simulink model "Lab1"  (R2016a)
settings: Solver=VariableStepAuto  StartTime=0.0  StopTime=10.0  RelTol=1e-3
settings Model: Creator=KamalEldeen  LastModifiedBy=KamalEldeen

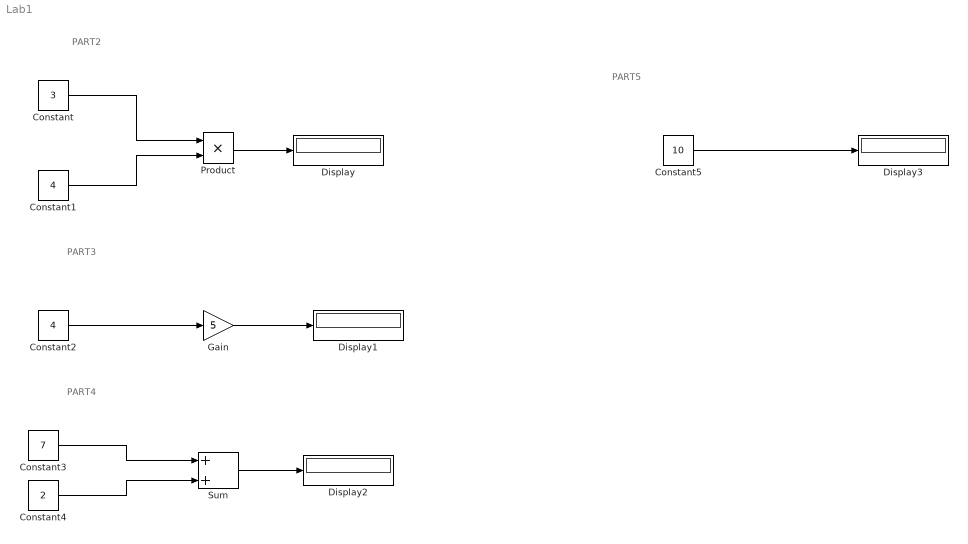
== system Lab1 ==
  note: PART2
  note: PART3
  note: PART4
  note: PART5
  Constant : Constant  Value=3
  Constant1 : Constant  Value=4
  Constant2 : Constant  Value=4
  Constant3 : Constant  Value=7
  Constant4 : Constant  Value=2
  Constant5 : Constant  Value=10
  Display{,1..3} (4 alike) : Display
  Gain : Gain  Gain=5
  Product : Product
  Sum : Sum
  wires:
  Constant/1 -> Product/1
  Constant1/1 -> Product/2
  Product/1 -> Display/1
  Gain/1 -> Display1/1
  Constant2/1 -> Gain/1
  Constant4/1 -> Sum/2
  Constant3/1 -> Sum/1
  Sum/1 -> Display2/1
  Constant5/1 -> Display3/1
